simulink model "stirred_tank_exotherm_start_R2018a"  (R2018a)
settings: Solver=VariableStepAuto  StartTime=0.0  StopTime=80  MaxStep=0.01  RelTol=1e-3
model workspace (MATLAB code in the model file):
  | gamma = 1;
  | a_A = 4;
  | a_T = 3;
  | x_init = 1;
  | a_c = 1;
  | a_cc = 2;
  | T_init = 1;
  | T_c_init = 1;
settings Model: Creator=kjartan  LastModifiedBy=kjartan
settings CodeAppCC: StateflowObjectComments=on

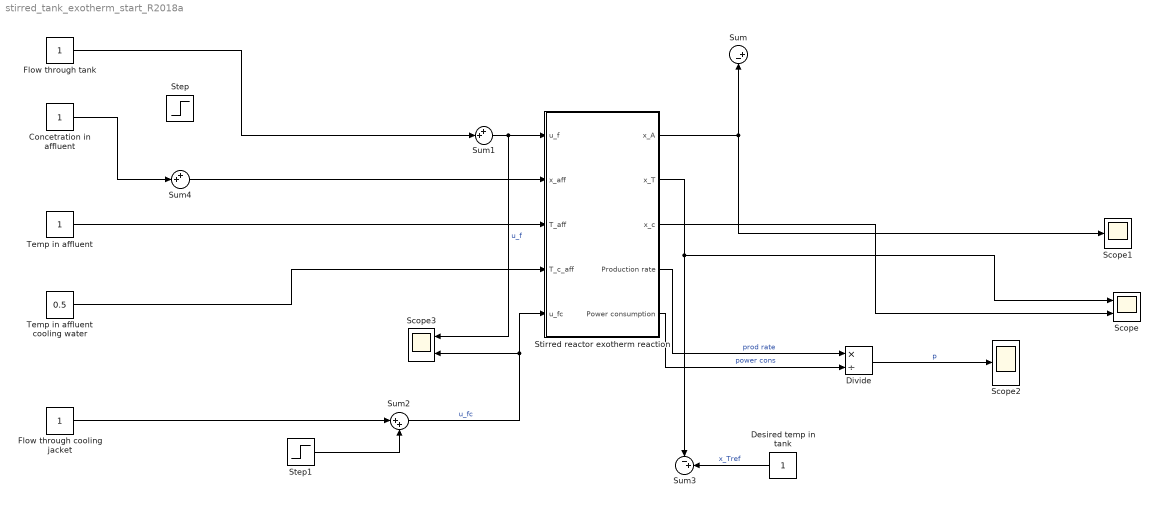
== system stirred_tank_exotherm_start_R2018a ==
  Concetration in affluent : Constant
  Desired temp in tank : Constant
  Divide : Product  Inputs=*/
  Flow through cooling jacket : Constant
  Flow through tank : Constant
  Scope : Scope  NumInputPorts=2
  Scope1 : Scope
  Scope2 : Scope
  Scope3 : Scope  NumInputPorts=2
  Step : Step  Time=40  After=0.2  SampleTime=0
  Step1 : Step  Time=40  After=0.2  SampleTime=0
  Stirred reactor exotherm reaction : Subsystem
  Sum : Sum  Inputs=|+-
  Sum1 : Sum  Inputs=++|
  Sum2 : Sum  Inputs=|++
  Sum3 : Sum  Inputs=-+|
  Sum4 : Sum  Inputs=++|
  Temp in affluent : Constant
  Temp in affluent cooling water : Constant  Value=0.5
  wires:
  Concetration in affluent/1 -> Sum4/2
  Temp in affluent cooling water/1 -> Stirred reactor exotherm reaction/4(T_c_aff)
  Stirred reactor exotherm reaction/2(x_T) -> Sum3/1, Scope/1
  Stirred reactor exotherm reaction/3(x_c) -> Scope/2
  Flow through cooling jacket/1 -> Sum2/1
  Flow through tank/1 -> Sum1/2
  Sum1/1 -> Stirred reactor exotherm reaction/1(u_f), Scope3/1  "u_f"
  Sum2/1 -> Stirred reactor exotherm reaction/5(u_fc), Scope3/2  "u_fc"
  Desired temp in tank/1 -> Sum3/2  "x_Tref"
  Sum4/1 -> Stirred reactor exotherm reaction/2(x_aff)
  Stirred reactor exotherm reaction/4(Production rate) -> Divide/1  "prod rate"
  Stirred reactor exotherm reaction/5(Power consumption) -> Divide/2  "power cons"
  Divide/1 -> Scope2/1  "p"
  Temp in affluent/1 -> Stirred reactor exotherm reaction/3(T_aff)
  ? -> Sum/1  "x_Aref"
  Stirred reactor exotherm reaction/1(x_A) -> Scope1/1, Sum/2
  Step1/1 -> Sum2/2

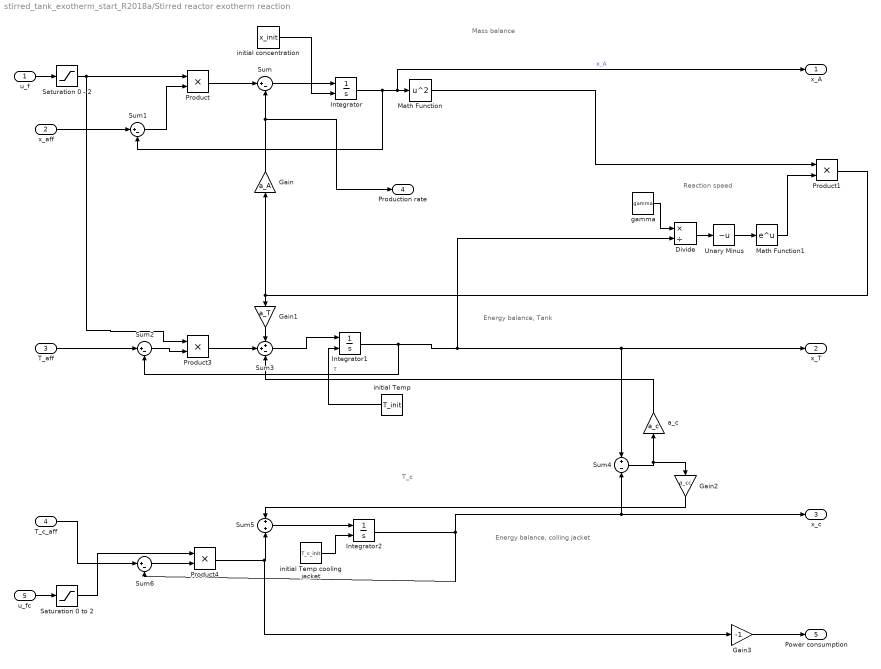
== system stirred_tank_exotherm_start_R2018a/Stirred reactor exotherm reaction ==
  note: Energy balance,
      | colling jacket
  note: Energy balance, Tank
  note: Reaction speed
  note: Mass balance
  note: T_c
  u_f : Inport
  x_aff : Inport  Port=2
  T_aff : Inport  Port=3
  T_c_aff : Inport  Port=4
  u_fc : Inport  Port=5
  Divide : Product  Inputs=*/
  Gain : Gain  Gain=a_A
  Gain1 : Gain  Gain=a_T
  Gain2 : Gain  Gain=a_cc
  Gain3 : Gain  Gain=-1
  Integrator : Integrator  InitialConditionSource=external
  Integrator1 : Integrator  InitialConditionSource=external
  Integrator2 : Integrator  InitialConditionSource=external
  Math Function : Math  Operator=square  SaturateOnIntegerOverflow=on
  Math Function1 : Math  SaturateOnIntegerOverflow=on
  Product{,1,3..4} (4 alike) : Product
  Saturation 0 - 2 : Saturate  UpperLimit=2  LowerLimit=0
  Saturation 0 to 2 : Saturate  UpperLimit=4  LowerLimit=0
  Sum{,1..2,6} (4 alike) : Sum  Inputs=|+-
  Sum3 : Sum  Inputs=++-
  Sum4 : Sum  Inputs=+|-
  Sum5 : Sum  Inputs=+|+
  Unary Minus : UnaryMinus
  a_c : Gain  Gain=a_c
  gamma : Constant  Value=gamma
  initial Temp : Constant  Value=T_init
  initial Temp cooling jacket : Constant  Value=T_c_init
  initial concentration : Constant  Value=x_init
  x_A : Outport  VectorParamsAs1DForOutWhenUnconnected=off
  x_T : Outport  Port=2  VectorParamsAs1DForOutWhenUnconnected=off
  x_c : Outport  Port=3  VectorParamsAs1DForOutWhenUnconnected=off
  Production rate : Outport  Port=4  VectorParamsAs1DForOutWhenUnconnected=off
  Power consumption : Outport  Port=5  VectorParamsAs1DForOutWhenUnconnected=off
  wires:
  Integrator/1 -> x_A/1, Math Function/1, Sum1/2  "x_A"
  initial Temp/1 -> Integrator1/2
  Product1/1 -> Gain/1, Gain1/1
  Unary Minus/1 -> Math Function1/1
  Sum2/1 -> Product3/2
  Integrator2/1 -> Sum4/2, x_c/1, Sum6/2
  Sum4/1 -> Gain2/1, a_c/1
  Sum5/1 -> Integrator2/1
  initial Temp cooling jacket/1 -> Integrator2/2
  Sum6/1 -> Product4/2
  T_c_aff/1 -> Sum6/1
  Math Function1/1 -> Product1/2
  u_f/1 -> Saturation 0 - 2/1
  Integrator1/1 -> Sum2/2, Divide/2, x_T/1, Sum4/1  "T"
  gamma/1 -> Divide/1
  Sum/1 -> Integrator/1
  Math Function/1 -> Product1/1
  Divide/1 -> Unary Minus/1
  T_aff/1 -> Sum2/1
  Sum3/1 -> Integrator1/1
  x_aff/1 -> Sum1/1
  initial concentration/1 -> Integrator/2
  Sum1/1 -> Product/2
  Gain/1 -> Production rate/1, Sum/2
  Gain1/1 -> Sum3/1
  Product3/1 -> Sum3/2
  u_fc/1 -> Saturation 0 to 2/1
  Product4/1 -> Gain3/1, Sum5/2
  a_c/1 -> Sum3/3
  Gain2/1 -> Sum5/1
  Saturation 0 - 2/1 -> Product3/1, Product/1
  Saturation 0 to 2/1 -> Product4/1
  Gain3/1 -> Power consumption/1
  Product/1 -> Sum/1
